simulink model "trim_sim"  (R2020b)
settings: Solver=VariableStepAuto  StartTime=0.0  StopTime=10.0  RelTol=1e-3  SampleTimeConstraint=STIndependent
undefined symbols (not defined in the file): Aircraft, Earth, Env, InitCond, WGS84
libraries: aerolibconvert2 x6, aerolibadyn x3, aerolibasang x3, aerolibatmos2 x1, sharedutil x1, aerolibbdyn x1, shared6dof x1, simulink x1, aerolibtransform2 x1, aerolibgravity2 x1
settings Model: Creator=brian  LastModifiedBy=brian

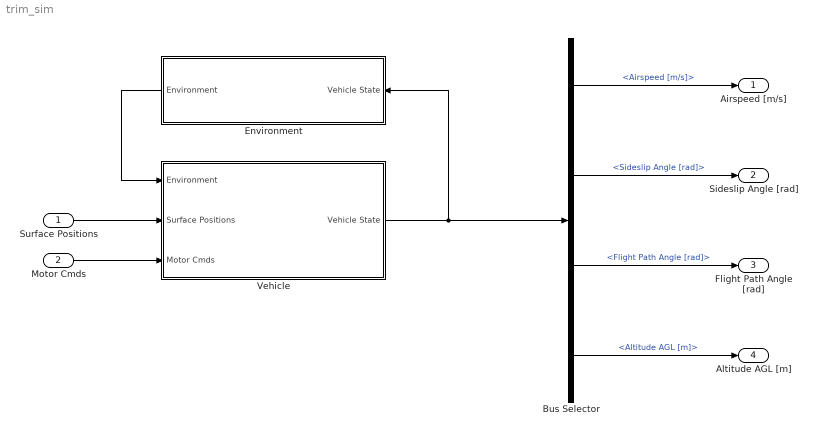
== system trim_sim ==
  Surface Positions : Inport
  Motor Cmds : Inport  Port=2  PortDimensions=Aircraft.Motor.nMotor
  Bus Selector : BusSelector  OutputSignals=Airspeed [m/s],Sideslip Angle [rad],Flight Path Angle [rad],Altitude AGL [m]
  Environment : Subsystem
  Vehicle : Subsystem
  Airspeed [m/s] : Outport
  Sideslip Angle [rad] : Outport  Port=2
  Flight Path Angle [rad] : Outport  Port=3
  Altitude AGL [m] : Outport  Port=4
  wires:
  Vehicle/1(Vehicle State) -> Environment/1(Vehicle State), Bus Selector/1
  Environment/1(Environment) -> Vehicle/1(Environment)
  Surface Positions/1 -> Vehicle/2(Surface Positions)
  Motor Cmds/1 -> Vehicle/3(Motor Cmds)
  Bus Selector/1 -> Airspeed [m/s]/1  "<Airspeed [m/s]>"
  Bus Selector/2 -> Sideslip Angle [rad]/1  "<Sideslip Angle [rad]>"
  Bus Selector/3 -> Flight Path Angle [rad]/1  "<Flight Path Angle [rad]>"
  Bus Selector/4 -> Altitude AGL [m]/1  "<Altitude AGL [m]>"

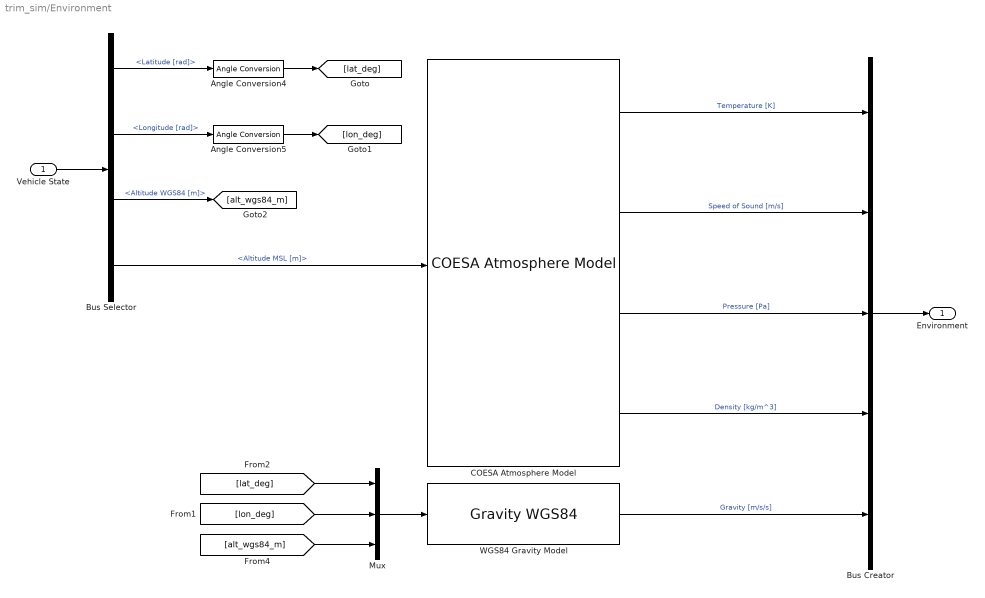
== system trim_sim/Environment ==
  Vehicle State : Inport
  Angle Conversion4 : aerolibconvert2/Angle Conversion  IU=rad  OU=deg
  Angle Conversion5 : aerolibconvert2/Angle Conversion  IU=rad  OU=deg
  Bus Creator : BusCreator  Inputs=5
  Bus Selector : BusSelector  OutputSignals=Latitude [rad],Longitude [rad],Altitude WGS84 [m],Altitude MSL [m]
  COESA Atmosphere Model : aerolibatmos2/COESA Atmosphere Model  units=Metric (MKS)  spec=1976 COESA-extended U.S. Standard Atmosphere  model=Profile  profile_var=High temperature  profile_percent=1%  profile_alt=5 km (16404 ft)  envelope_var=High temperature  envelope_percent=1%  action=Warning
  Mux : Mux  Inputs=3
  "WGS84 Gravity Model  " : GravityWGS84
  Environment : Outport
  wires:
  Vehicle State/1 -> Bus Selector/1
  Bus Selector/1 -> Angle Conversion4/1  "<Latitude [rad]>"
  Bus Selector/2 -> Angle Conversion5/1  "<Longitude [rad]>"
  Bus Selector/3 -> [alt_wgs84_m]  "<Altitude WGS84 [m]>"
  Bus Creator/1 -> Environment/1
  COESA Atmosphere Model/3 -> Bus Creator/3  "Pressure [Pa]"
  COESA Atmosphere Model/2 -> Bus Creator/2  "Speed of Sound [m/s]"
  COESA Atmosphere Model/1 -> Bus Creator/1  "Temperature [K]"
  COESA Atmosphere Model/4 -> Bus Creator/4  "Density [kg/m^3]"
  "WGS84 Gravity Model  "/1 -> Bus Creator/5  "Gravity [m/s/s]"
  Bus Selector/4 -> COESA Atmosphere Model/1  "<Altitude MSL [m]>"
  Mux/1 -> "WGS84 Gravity Model  "/1
  Angle Conversion4/1 -> [lat_deg]
  Angle Conversion5/1 -> [lon_deg]
  [alt_wgs84_m] -> Mux/3
  [lon_deg] -> Mux/2
  [lat_deg] -> Mux/1

== system trim_sim/Vehicle ==
  Environment : Inport
  Surface Positions : Inport  Port=2  PortDimensions=Aircraft.Surf.nSurf
  Motor Cmds : Inport  Port=3
  Bus Creator : BusCreator  Inputs=25
  Bus Selector : BusSelector  OutputSignals=Gravity [m/s/s],Density [kg/m^3],Speed of Sound [m/s]
  Bus Selector1 : BusSelector  OutputSignals=Body Velocity [m/s],Body Rotational Rate [rad/s],Dynamic Pressure [Pa],Airspeed [m/s],Angle of Attack [rad],Sideslip Angle [rad],DCM_be
  Forces and Moments : Subsystem
  Vehicle Model : Subsystem
  Vehicle State : Outport
  wires:
  Surface Positions/1 -> Forces and Moments/8(Surface Positions [rad])
  Environment/1 -> Bus Selector/1
  Bus Creator/1 -> Bus Selector1/1, Vehicle State/1
  Motor Cmds/1 -> Forces and Moments/9(Motor Cmds)
  Vehicle Model/1(Latitude [rad]) -> Bus Creator/1  "Latitude [rad]"
  Vehicle Model/2(Longitude [rad]) -> Bus Creator/2  "Longitude [rad]"
  Vehicle Model/3(Altitude WGS84 [m]) -> Bus Creator/3  "Altitude WGS84 [m]"
  Vehicle Model/4(Altitude MSL [m]) -> Bus Creator/4  "Altitude MSL [m]"
  Vehicle Model/5(Altitude AGL [m]) -> Bus Creator/5  "Altitude AGL [m]"
  Vehicle Model/6(NED Position [m]) -> Bus Creator/6  "NED Position [m]"
  Vehicle Model/7(NED Velocity [m/s]) -> Bus Creator/7  "NED Velocity [m/s]"
  Vehicle Model/8(NED Accel [m/s/s]) -> Bus Creator/8  "NED Accel [m/s/s]"
  Vehicle Model/9(Pitch [rad]) -> Bus Creator/9  "Pitch [rad]"
  Vehicle Model/10(Roll [rad]) -> Bus Creator/10  "Roll [rad]"
  Vehicle Model/11(Yaw [rad]) -> Bus Creator/11  "Yaw [rad]"
  Vehicle Model/12(Body Velocity [m/s]) -> Bus Creator/12  "Body Velocity [m/s]"
  Vehicle Model/13(Body Accel [m/s/s]) -> Bus Creator/13  "Body Accel [m/s/s]"
  Vehicle Model/14(Body Rotational Rate [rad/s]) -> Bus Creator/14  "Body Rotational Rate [rad/s]"
  Vehicle Model/15(Body Rotational Accel [rad/s/s]) -> Bus Creator/15  "Body Rotational Accel [rad/s/s]"
  Vehicle Model/16(Dynamic Pressure [Pa]) -> Bus Creator/16  "Dynamic Pressure [Pa]"
  Vehicle Model/17(Airspeed [m/s]) -> Bus Creator/17  "Airspeed [m/s]"
  Vehicle Model/18(Mach) -> Bus Creator/18  "Mach"
  Vehicle Model/19(Angle of Attack [rad]) -> Bus Creator/19  "Angle of Attack [rad]"
  Vehicle Model/20(Angle of Attack Rate [rad/s]) -> Bus Creator/20  "Angle of Attack Rate [rad/s]"
  Vehicle Model/21(Sideslip Angle [rad]) -> Bus Creator/21  "Sideslip Angle [rad]"
  Vehicle Model/22(Sideslip Angle Rate [rad/s]) -> Bus Creator/22  "Sideslip Angle Rate [rad/s]"
  Vehicle Model/23(Ground Track [rad]) -> Bus Creator/23  "Ground Track [rad]"
  Vehicle Model/24(Flight Path Angle [rad]) -> Bus Creator/24  "Flight Path Angle [rad]"
  Vehicle Model/25(DCM_be) -> Bus Creator/25  "DCM_be"
  Bus Selector1/7 -> Forces and Moments/7(DCM_be)  "<DCM_be>"
  Bus Selector1/6 -> Forces and Moments/6(Sideslip Angle [rad])  "<Sideslip Angle [rad]>"
  Bus Selector1/5 -> Forces and Moments/5(Angle of Attack [rad])  "<Angle of Attack [rad]>"
  Bus Selector1/4 -> Forces and Moments/4(Airspeed [m/s])  "<Airspeed [m/s]>"
  Bus Selector1/3 -> Forces and Moments/3(Dynamic Pressure [Pa])  "<Dynamic Pressure [Pa]>"
  Bus Selector1/2 -> Forces and Moments/2(Body Rotational Rate [rad/s])  "<Body Rotational Rate [rad/s]>"
  Bus Selector1/1 -> Forces and Moments/1(Body Velocity [m/s])  "<Body Velocity [m/s]>"
  Bus Selector/1 -> Forces and Moments/10(Gravity [m/s/s])  "<Gravity [m/s/s]>"
  Bus Selector/2 -> Forces and Moments/11(Density [kg/m^3]), Vehicle Model/3(Density [kg/m^3])  "<Density [kg/m^3]>"
  Bus Selector/3 -> Vehicle Model/4(Speed of Sound [m/s])  "<Speed of Sound [m/s]>"
  Forces and Moments/1(Fxyz [N]) -> Vehicle Model/1(Fxyz [N])
  Forces and Moments/2(Mxyz [N-m]) -> Vehicle Model/2(Mxyz [N-m])

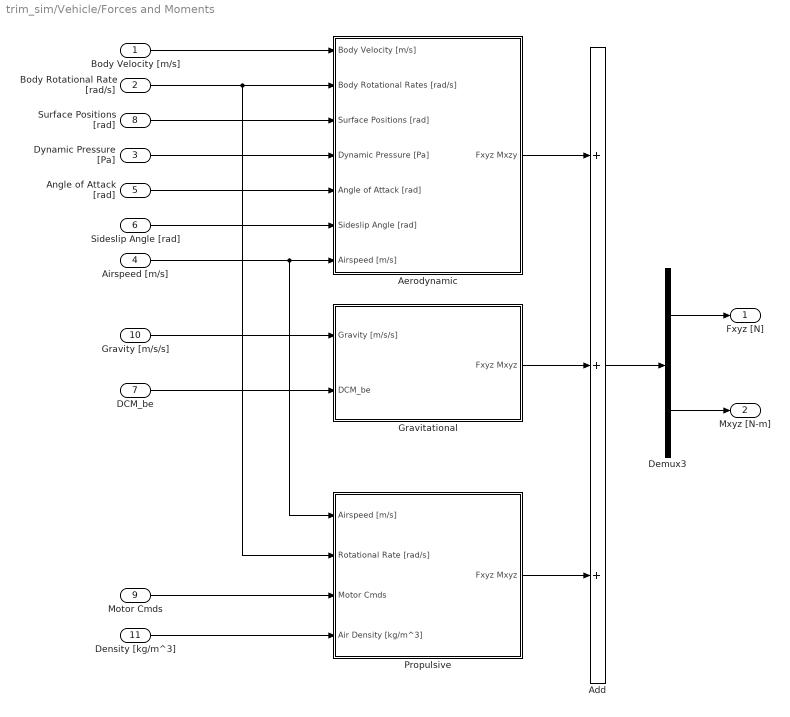
== system trim_sim/Vehicle/Forces and Moments ==
  Body Velocity [m/s] : Inport
  Body Rotational Rate [rad/s] : Inport  Port=2
  Dynamic Pressure [Pa] : Inport  Port=3
  Airspeed [m/s] : Inport  Port=4
  Angle of Attack [rad] : Inport  Port=5
  Sideslip Angle [rad] : Inport  Port=6
  DCM_be : Inport  Port=7
  Surface Positions [rad] : Inport  Port=8
  Motor Cmds : Inport  Port=9
  Gravity [m/s/s] : Inport  Port=10
  Density [kg/m^3] : Inport  Port=11
  Add : Sum  Inputs=+++
  Aerodynamic : Subsystem
  Demux3 : Demux  Outputs=2
  Gravitational : Subsystem
  Propulsive : Subsystem
  Fxyz [N] : Outport
  Mxyz [N-m] : Outport  Port=2
  wires:
  Propulsive/1(Fxyz Mxyz) -> Add/3
  Density [kg/m^3]/1 -> Propulsive/4(Air Density [kg/m^3])
  Motor Cmds/1 -> Propulsive/3(Motor Cmds)
  Add/1 -> Demux3/1
  Demux3/2 -> Mxyz [N-m]/1
  Aerodynamic/1(Fxyz Mxzy) -> Add/1
  Demux3/1 -> Fxyz [N]/1
  Body Rotational Rate [rad/s]/1 -> Propulsive/2(Rotational Rate [rad/s]), Aerodynamic/2(Body Rotational Rates [rad/s])
  DCM_be/1 -> Gravitational/2(DCM_be)
  Angle of Attack [rad]/1 -> Aerodynamic/5(Angle of Attack [rad])
  Gravitational/1(Fxyz Mxyz) -> Add/2
  Sideslip Angle [rad]/1 -> Aerodynamic/6(Sideslip Angle [rad])
  Body Velocity [m/s]/1 -> Aerodynamic/1(Body Velocity [m/s])
  Dynamic Pressure [Pa]/1 -> Aerodynamic/4(Dynamic Pressure [Pa])
  Airspeed [m/s]/1 -> Propulsive/1(Airspeed [m/s]), Aerodynamic/7(Airspeed [m/s])
  Gravity [m/s/s]/1 -> Gravitational/1(Gravity [m/s/s])
  Surface Positions [rad]/1 -> Aerodynamic/3(Surface Positions [rad])

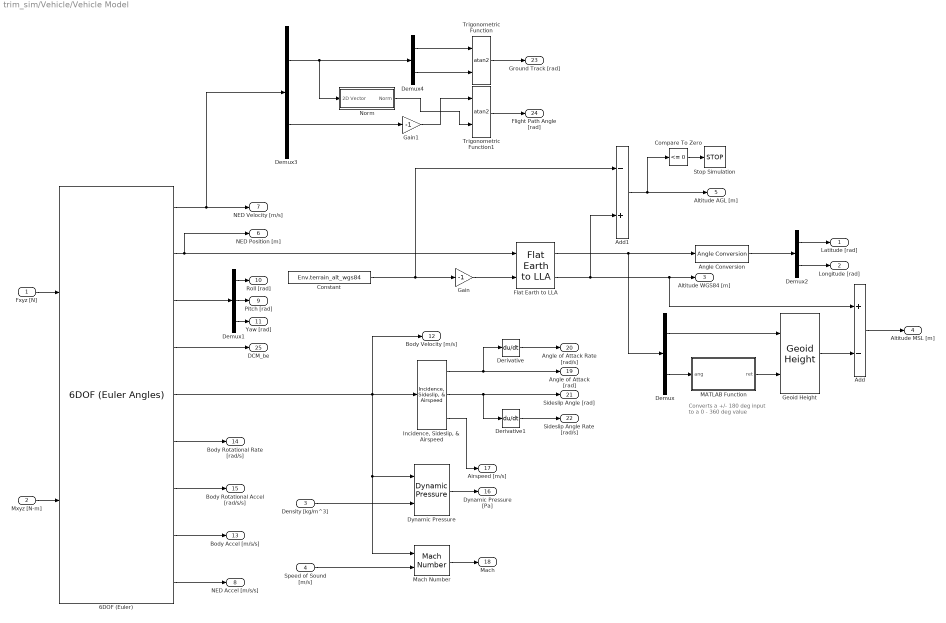
== system trim_sim/Vehicle/Vehicle Model ==
  note: Converts a +/- 180 deg
      | input to a 0 - 360 deg value
  Fxyz [N] : Inport
  Mxyz [N-m] : Inport  Port=2
  Density [kg/m^3] : Inport  Port=3
  Speed of Sound [m/s] : Inport  Port=4
  6DOF (Euler) : shared6dof/6DOF (Euler Angles)  units=Metric (MKS)  mtype=Fixed  rep=Euler Angles  xme_0=InitCond.ned_pos_m  Vm_0=InitCond.body_vel_mps  eul_0=InitCond.euler_rad  pm_0=InitCond.body_rot_rate_radps  mass_0=Aircraft.Mass.mass_kg  mass_e=0.5  mass_f=2.0  inertia=Aircraft.Mass.inertia_kgm2  inertia_e=eye(3)  inertia_f=2*eye(3)  k_quat=1.0  vre_flag=on  abi_flag=on  aMode=0  xme_statename=''  Vm_statename=''  eul_statename=''  quat_statename=''  pm_statename=''  mass_statename=''
      settings: SourceProductBaseCode=AE,PW,MT,UV,VE,VP
  Add : Sum  Inputs=+-
  Add1 : Sum  Inputs=-+
  Angle Conversion : aerolibconvert2/Angle Conversion  IU=deg  OU=rad
  Compare To Zero : simulink/Logic and Bit Operations/Compare To Zero  relop=<=  OutDataTypeStr=boolean
  Constant : Constant  Value=Env.terrain_alt_wgs84
  Demux : Demux  Outputs=2
  Demux1 : Demux  Outputs=3
  Demux2 : Demux  Outputs=2
  Demux3 : Demux  Outputs=[2 1]
  Demux4 : Demux  Outputs=2
  Derivative : Derivative
  Derivative1 : Derivative
  Dynamic Pressure : aerolibasang/Dynamic Pressure
  Flat Earth to LLA : aerolibtransform2/Flat Earth to LLA  units=Metric (MKS)  ptype=Earth (WGS84)  F=1/298.257223563  R=6378137  refPosPort=off  LL0=[rad2deg(InitCond.lat_rad) rad2deg(InitCond.lon_rad)]  psi=0
  Gain : Gain  Gain=-1
  Gain1 : Gain  Gain=-1
  Geoid Height : aerolibgravity2/Geoid Height  units=Metric (MKS)  gtype=EGM2008  datafile='geoidegm96grid'  dtype=double  action=Warning
      settings: SourceProductBaseCode=AE
  "Incidence, Sideslip, & Airspeed" : aerolibasang/Incidence, Sideslip, & Airspeed
  MATLAB Function : MATLAB Function  TreatAsAtomicUnit=on
  Mach Number : aerolibasang/Mach Number
      settings: SourceProductBaseCode=AE
  Norm : Subsystem
  Stop Simulation : Stop
  Trigonometric Function : Trigonometry  Operator=atan2
  Trigonometric Function1 : Trigonometry  Operator=atan2
  Latitude [rad] : Outport
  Longitude [rad] : Outport  Port=2
  Altitude WGS84 [m] : Outport  Port=3
  Altitude MSL [m] : Outport  Port=4
  Altitude AGL [m] : Outport  Port=5
  NED Position [m] : Outport  Port=6
  NED Velocity [m/s] : Outport  Port=7
  NED Accel [m/s/s] : Outport  Port=8
  Pitch [rad] : Outport  Port=9
  Roll [rad] : Outport  Port=10
  Yaw [rad] : Outport  Port=11
  Body Velocity [m/s] : Outport  Port=12
  Body Accel [m/s/s] : Outport  Port=13
  Body Rotational Rate [rad/s] : Outport  Port=14
  Body Rotational Accel [rad/s/s] : Outport  Port=15
  Dynamic Pressure [Pa] : Outport  Port=16
  Airspeed [m/s] : Outport  Port=17
  Mach : Outport  Port=18
  Angle of Attack [rad] : Outport  Port=19
  Angle of Attack Rate [rad/s] : Outport  Port=20
  Sideslip Angle [rad] : Outport  Port=21
  Sideslip Angle Rate [rad/s] : Outport  Port=22
  Ground Track [rad] : Outport  Port=23
  Flight Path Angle [rad] : Outport  Port=24
  DCM_be : Outport  Port=25
  wires:
  Fxyz [N]/1 -> 6DOF (Euler)/1
  Mxyz [N-m]/1 -> 6DOF (Euler)/2
  6DOF (Euler)/5 -> Body Velocity [m/s]/1, "Incidence, Sideslip, & Airspeed"/1, Dynamic Pressure/1, Mach Number/1
  Flat Earth to LLA/1 -> Demux/1, Angle Conversion/1
  Flat Earth to LLA/2 -> Add1/2, Add/1, Altitude WGS84 [m]/1
  Geoid Height/1 -> Add/2
  Demux/2 -> MATLAB Function/1(ang)
  Demux/1 -> Geoid Height/1
  "Incidence, Sideslip, & Airspeed"/3 -> Airspeed [m/s]/1
  Density [kg/m^3]/1 -> Dynamic Pressure/2
  Angle Conversion/1 -> Demux2/1
  6DOF (Euler)/4 -> DCM_be/1
  Demux1/1 -> Roll [rad]/1
  6DOF (Euler)/3 -> Demux1/1
  Demux1/2 -> Pitch [rad]/1
  Demux1/3 -> Yaw [rad]/1
  Dynamic Pressure/1 -> Dynamic Pressure [Pa]/1
  "Incidence, Sideslip, & Airspeed"/1 -> Derivative/1, Angle of Attack [rad]/1
  "Incidence, Sideslip, & Airspeed"/2 -> Derivative1/1, Sideslip Angle [rad]/1
  Add/1 -> Altitude MSL [m]/1
  Gain/1 -> Flat Earth to LLA/2
  Demux2/2 -> Longitude [rad]/1
  Demux2/1 -> Latitude [rad]/1
  6DOF (Euler)/2 -> NED Position [m]/1, Flat Earth to LLA/1
  6DOF (Euler)/6 -> Body Rotational Rate [rad/s]/1
  6DOF (Euler)/7 -> Body Rotational Accel [rad/s/s]/1
  6DOF (Euler)/8 -> Body Accel [m/s/s]/1
  6DOF (Euler)/1 -> Demux3/1, NED Velocity [m/s]/1
  MATLAB Function/1(ret) -> Geoid Height/2
  Demux3/1 -> Norm/1(2D Vector), Demux4/1
  Demux4/1 -> Trigonometric Function/1
  Demux4/2 -> Trigonometric Function/2
  Trigonometric Function/1 -> Ground Track [rad]/1
  Demux3/2 -> Gain1/1
  Gain1/1 -> Trigonometric Function1/1
  Norm/1(Norm) -> Trigonometric Function1/2
  Trigonometric Function1/1 -> Flight Path Angle [rad]/1
  6DOF (Euler)/9 -> NED Accel [m/s/s]/1
  Speed of Sound [m/s]/1 -> Mach Number/2
  Mach Number/1 -> Mach/1
  Derivative/1 -> Angle of Attack Rate [rad/s]/1
  Derivative1/1 -> Sideslip Angle Rate [rad/s]/1
  Constant/1 -> Add1/1, Gain/1
  Add1/1 -> Compare To Zero/1, Altitude AGL [m]/1
  Compare To Zero/1 -> Stop Simulation/1

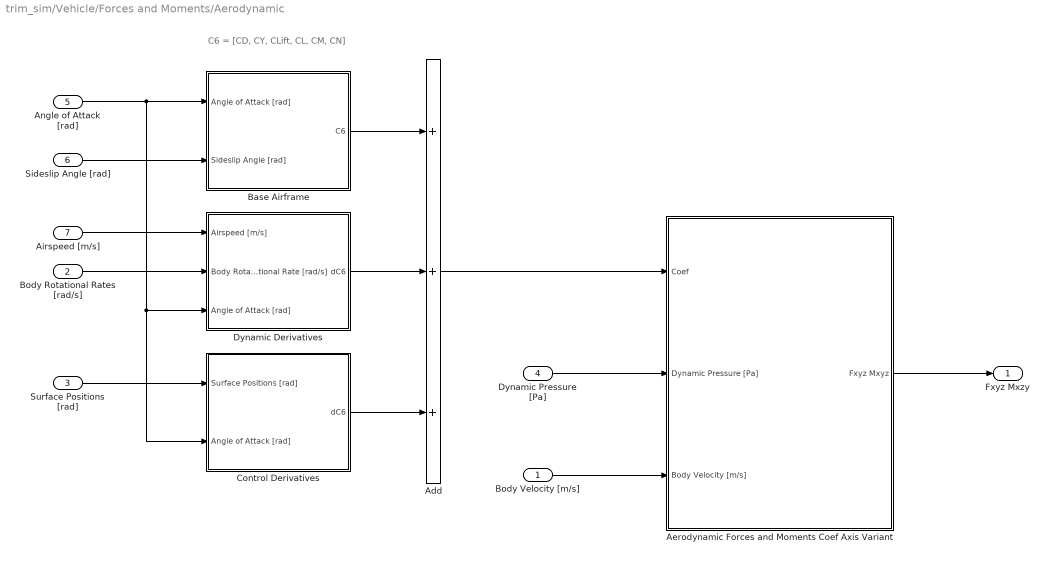
== system trim_sim/Vehicle/Forces and Moments/Aerodynamic ==
  note: C6 = [CD, CY, CLift, CL, CM, CN]
  Body Velocity [m/s] : Inport
  Body Rotational Rates [rad/s] : Inport  Port=2
  Surface Positions [rad] : Inport  Port=3
  Dynamic Pressure [Pa] : Inport  Port=4
  Angle of Attack [rad] : Inport  Port=5
  Sideslip Angle [rad] : Inport  Port=6
  Airspeed [m/s] : Inport  Port=7
  Add : Sum  Inputs=+++
  Aerodynamic Forces and Moments Coef Axis Variant : Subsystem  Variant=on
  Base Airframe : Subsystem
  Control Derivatives : Subsystem
  Dynamic Derivatives : Subsystem
  Fxyz Mxzy : Outport
  wires:
  Base Airframe/1(C6) -> Add/1
  Dynamic Derivatives/1(dC6) -> Add/2
  Sideslip Angle [rad]/1 -> Base Airframe/2(Sideslip Angle [rad])
  Angle of Attack [rad]/1 -> Base Airframe/1(Angle of Attack [rad]), Control Derivatives/2(Angle of Attack [rad]), Dynamic Derivatives/3(Angle of Attack [rad])
  Body Rotational Rates [rad/s]/1 -> Dynamic Derivatives/2(Body Rotational Rate [rad/s])
  Airspeed [m/s]/1 -> Dynamic Derivatives/1(Airspeed [m/s])
  Surface Positions [rad]/1 -> Control Derivatives/1(Surface Positions [rad])
  Control Derivatives/1(dC6) -> Add/3
  Add/1 -> Aerodynamic Forces and Moments Coef Axis Variant/1(Coef)
  Body Velocity [m/s]/1 -> Aerodynamic Forces and Moments Coef Axis Variant/3(Body Velocity [m/s])
  Dynamic Pressure [Pa]/1 -> Aerodynamic Forces and Moments Coef Axis Variant/2(Dynamic Pressure [Pa])
  Aerodynamic Forces and Moments Coef Axis Variant/1(Fxyz Mxyz) -> Fxyz Mxzy/1

== system trim_sim/Vehicle/Forces and Moments/Gravitational ==
  Gravity [m/s/s] : Inport
  DCM_be : Inport  Port=2
  Gravity Moment : Constant  Value=[0 0 0]
  Mux : Mux  Inputs=2
  Product : Product
  Product1 : Product  Multiplication=Matrix(*)
  Reshape : Reshape  OutputDimensionality=Column vector (2-D)
  Reshape1 : Reshape
  UAV Mass : Constant  Value=Aircraft.Mass.mass_kg
  Fxyz Mxyz : Outport
  wires:
  UAV Mass/1 -> Product/2
  Product/1 -> Product1/2  "Gravity Force NED [N]"
  DCM_be/1 -> Product1/1
  Gravity Moment/1 -> Mux/2
  Mux/1 -> Fxyz Mxyz/1
  Reshape/1 -> Product/1
  Gravity [m/s/s]/1 -> Reshape/1
  Reshape1/1 -> Mux/1
  Product1/1 -> Reshape1/1  "Gravity Force Body [N]"

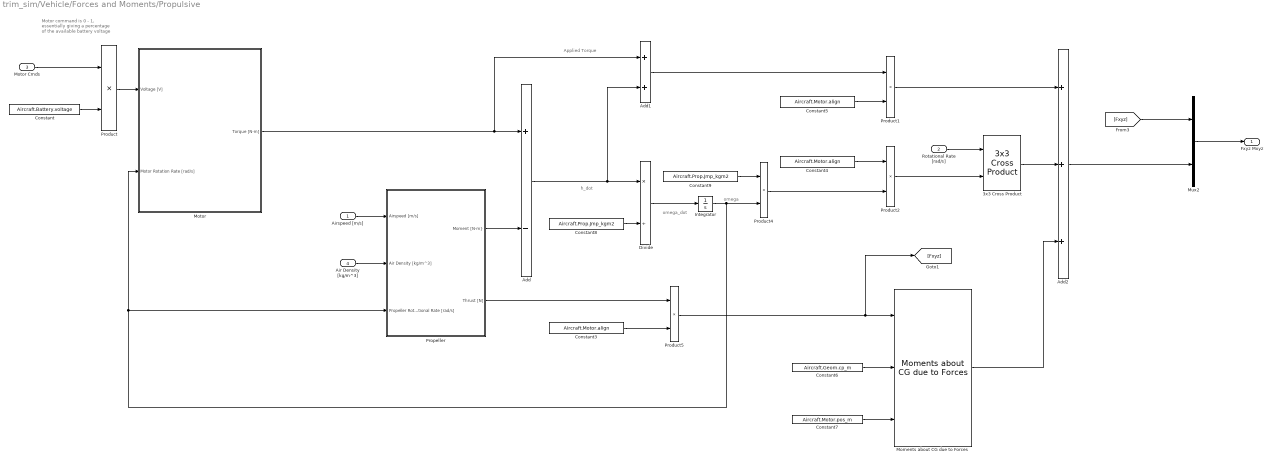
== system trim_sim/Vehicle/Forces and Moments/Propulsive ==
  note: Applied Torque
  note: omega
  note: Motor command is 0 - 1,
      | essentially giving a percentage
      | of the available battery voltage
  note: omega_dot
  note: h_dot
  Airspeed [m/s] : Inport
  Rotational Rate [rad/s] : Inport  Port=2
  Motor Cmds : Inport  Port=3
  Air Density [kg/m^3] : Inport  Port=4
  3x3 Cross Product : sharedutil/3x3 Cross Product  aMode=aMode
      settings: SourceProductBaseCode=AE,PW,MT,UV,VE,VP
  Add : Sum  Inputs=+-
  Add1 : Sum
  Add2 : Sum  Inputs=+++
  Constant : Constant  Value=Aircraft.Battery.voltage
  Constant3 : Constant  Value=Aircraft.Motor.align
  Constant4 : Constant  Value=Aircraft.Motor.align
  Constant5 : Constant  Value=Aircraft.Motor.align
  Constant6 : Constant  Value=Aircraft.Geom.cp_m
  Constant7 : Constant  Value=Aircraft.Motor.pos_m
  Constant8 : Constant  Value=Aircraft.Prop.Jmp_kgm2
  Constant9 : Constant  Value=Aircraft.Prop.Jmp_kgm2
  Divide : Product  Inputs=*/
  Integrator : Integrator  InitialCondition=InitCond.engine_speed_radps
  Moments about CG due to Forces : aerolibbdyn/Moments about CG  due to Forces
      settings: SourceProductBaseCode=AE
  Motor : Subsystem
  Mux2 : Mux  Inputs=2
  Product{,1..2,4..5} (5 alike) : Product
  Propeller : Subsystem
  Fxyz Mxyz : Outport
  wires:
  Divide/1 -> Integrator/1
  Constant3/1 -> Product5/2
  Constant8/1 -> Divide/2
  Product5/1 -> [Fxyz], Moments about CG due to Forces/1
  Product2/1 -> 3x3 Cross Product/2
  Product4/1 -> Product2/2
  Air Density [kg/m^3]/1 -> Propeller/2(Air Density [kg/m^3])
  Rotational Rate [rad/s]/1 -> 3x3 Cross Product/1
  Constant6/1 -> Moments about CG due to Forces/2
  Add/1 -> Add1/2, Divide/1
  Constant/1 -> Product/2
  Constant7/1 -> Moments about CG due to Forces/3
  Add1/1 -> Product1/1
  Product/1 -> Motor/1(Voltage [V])
  Constant5/1 -> Product1/2
  Propeller/2(Thrust [N]) -> Product5/1
  Integrator/1 -> Product4/2, Propeller/3(Propeller Rotational Rate [rad/s]), Motor/2(Motor Rotation Rate [rad/s])
  Airspeed [m/s]/1 -> Propeller/1(Airspeed [m/s])
  Moments about CG due to Forces/1 -> Add2/3
  Add2/1 -> Mux2/2
  3x3 Cross Product/1 -> Add2/2
  Mux2/1 -> Fxyz Mxyz/1
  Motor Cmds/1 -> Product/1
  [Fxyz] -> Mux2/1
  Propeller/1("Moment [N-m}") -> Add/2
  Constant4/1 -> Product2/1
  Motor/1(Torque [N-m]) -> Add1/1, Add/1
  Product1/1 -> Add2/1
  Constant9/1 -> Product4/1

== system trim_sim/Vehicle/Vehicle Model/Norm ==
  2D Vector : Inport
  Product : Product
  Sqrt : Sqrt  SaturateOnIntegerOverflow=on
  Sum of Elements : Sum  Inputs=+
  Norm : Outport
  wires:
  2D Vector/1 -> Product/2, Product/1
  Product/1 -> Sum of Elements/1
  Sum of Elements/1 -> Sqrt/1
  Sqrt/1 -> Norm/1

== system trim_sim/Vehicle/Forces and Moments/Aerodynamic/Aerodynamic Forces and Moments Coef Axis Variant ==
  Coef : Inport
  Dynamic Pressure [Pa] : Inport  Port=2
  Body Velocity [m/s] : Inport  Port=3
  Body Axis Coef : Subsystem  VariantControl=Aircraft.Aero.axis == 3
  Stability Axis Coef : Subsystem  VariantControl=Aircraft.Aero.axis == 2
  Wind Axis Coef : Subsystem  VariantControl=Aircraft.Aero.axis == 1
  Fxyz Mxyz : Outport

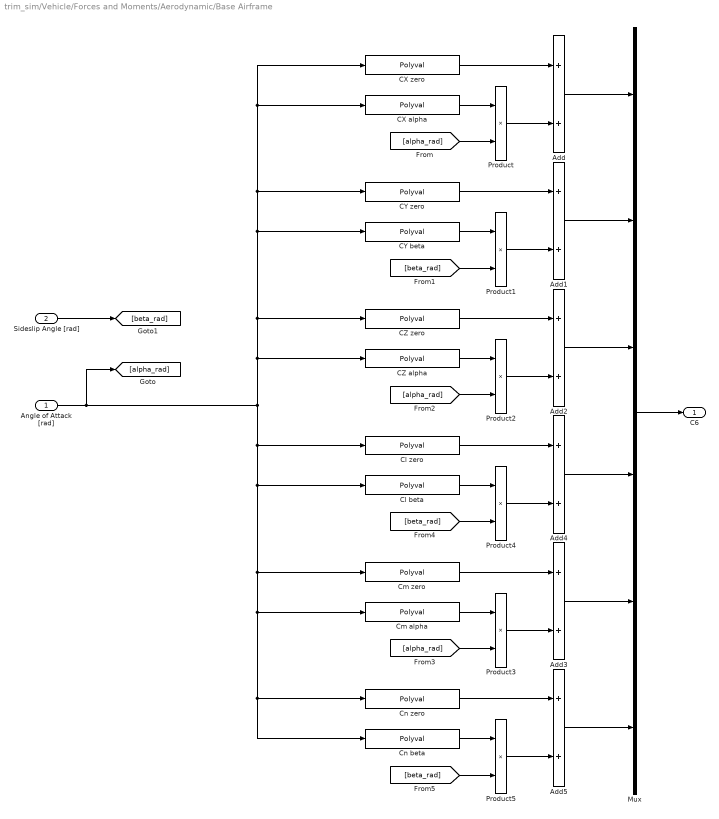
== system trim_sim/Vehicle/Forces and Moments/Aerodynamic/Base Airframe ==
  Angle of Attack [rad] : Inport
  Sideslip Angle [rad] : Inport  Port=2
  Add{,1..5} (6 alike) : Sum
  CX alpha : Polyval  Coefs=Aircraft.Aero.CX.alpha
  CX zero : Polyval  Coefs=Aircraft.Aero.CX.zero
  CY beta : Polyval  Coefs=Aircraft.Aero.CY.beta
  CY zero : Polyval  Coefs=Aircraft.Aero.CY.zero
  CZ alpha : Polyval  Coefs=Aircraft.Aero.CZ.alpha
  CZ zero : Polyval  Coefs=Aircraft.Aero.CZ.zero
  Cl beta : Polyval  Coefs=Aircraft.Aero.Cl.beta
  Cl zero : Polyval  Coefs=Aircraft.Aero.Cl.zero
  Cm alpha : Polyval  Coefs=Aircraft.Aero.Cm.alpha
  Cm zero : Polyval  Coefs=Aircraft.Aero.Cm.zero
  Cn beta : Polyval  Coefs=Aircraft.Aero.Cn.beta
  Cn zero : Polyval  Coefs=Aircraft.Aero.Cn.zero
  Mux : Mux  Inputs=6
  Product{,1..5} (6 alike) : Product
  C6 : Outport
  wires:
  Product/1 -> Add/2
  Add/1 -> Mux/1
  CX alpha/1 -> Product/1
  CX zero/1 -> Add/1
  Sideslip Angle [rad]/1 -> [beta_rad]
  [alpha_rad] -> Product/2
  Mux/1 -> C6/1
  [beta_rad] -> Product1/2
  CY zero/1 -> Add1/1
  CY beta/1 -> Product1/1
  Product1/1 -> Add1/2
  Add1/1 -> Mux/2
  CZ zero/1 -> Add2/1
  CZ alpha/1 -> Product2/1
  Add2/1 -> Mux/3
  Product2/1 -> Add2/2
  Product3/1 -> Add3/2
  Add3/1 -> Mux/5
  Cm alpha/1 -> Product3/1
  Cm zero/1 -> Add3/1
  [alpha_rad] -> Product2/2
  [alpha_rad] -> Product3/2
  Add4/1 -> Mux/4
  Product4/1 -> Add4/2
  Cl beta/1 -> Product4/1
  Cl zero/1 -> Add4/1
  [beta_rad] -> Product4/2
  [beta_rad] -> Product5/2
  Cn zero/1 -> Add5/1
  Cn beta/1 -> Product5/1
  Product5/1 -> Add5/2
  Add5/1 -> Mux/6
  Angle of Attack [rad]/1 -> [alpha_rad], Cl zero/1, Cl beta/1, Cm zero/1, Cm alpha/1, Cn zero/1, Cn beta/1, CZ alpha/1, CZ zero/1, CY beta/1, CY zero/1, CX alpha/1, CX zero/1

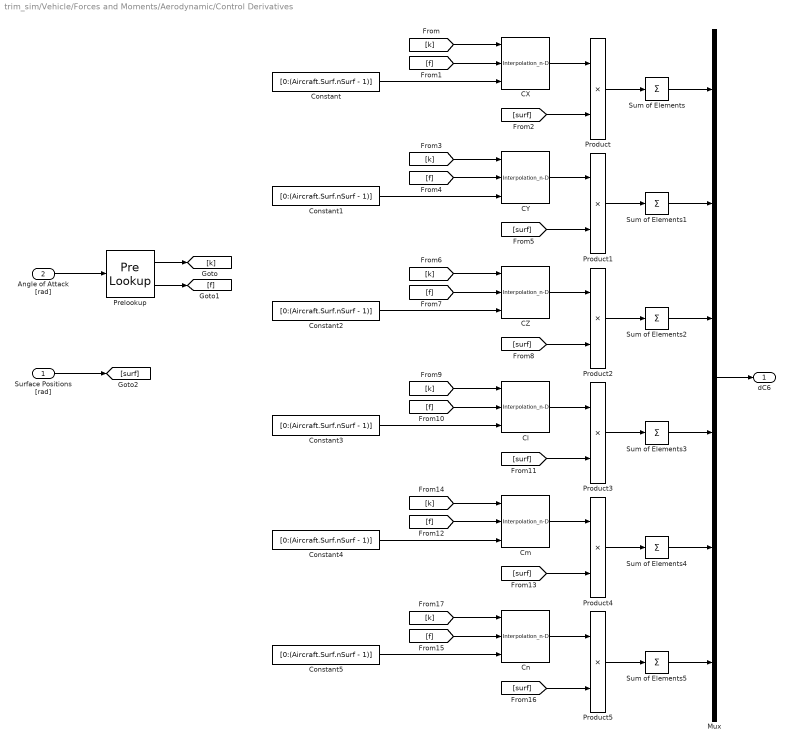
== system trim_sim/Vehicle/Forces and Moments/Aerodynamic/Control Derivatives ==
  Surface Positions [rad] : Inport
  Angle of Attack [rad] : Inport  Port=2
  CX : Interpolation_n-D  Table=Aircraft.Aero.CX.surf  DiagnosticForOutOfRangeInput=Warning  NumSelectionDims=1  InternalRulePriority=Speed
      settings: InputPortMap=u0,u1,u2
  CY : Interpolation_n-D  Table=Aircraft.Aero.CY.surf  DiagnosticForOutOfRangeInput=Warning  NumSelectionDims=1  InternalRulePriority=Speed
      settings: InputPortMap=u0,u1,u2
  CZ : Interpolation_n-D  Table=Aircraft.Aero.CZ.surf  DiagnosticForOutOfRangeInput=Warning  NumSelectionDims=1  InternalRulePriority=Speed
      settings: InputPortMap=u0,u1,u2
  Cl : Interpolation_n-D  Table=Aircraft.Aero.Cl.surf  DiagnosticForOutOfRangeInput=Warning  NumSelectionDims=1  InternalRulePriority=Speed
      settings: InputPortMap=u0,u1,u2
  Cm : Interpolation_n-D  Table=Aircraft.Aero.Cm.surf  DiagnosticForOutOfRangeInput=Warning  NumSelectionDims=1  InternalRulePriority=Speed
      settings: InputPortMap=u0,u1,u2
  Cn : Interpolation_n-D  Table=Aircraft.Aero.Cn.surf  DiagnosticForOutOfRangeInput=Warning  NumSelectionDims=1  InternalRulePriority=Speed
      settings: InputPortMap=u0,u1,u2
  Constant{,1..5} (6 alike) : Constant  Value=[0:(Aircraft.Surf.nSurf - 1)]
  Mux : Mux  Inputs=6
  Prelookup : PreLookup  BreakpointsData=Aircraft.Aero.CntrlEff.alpha  ExtrapMethod=Linear
  Product{,1..5} (6 alike) : Product
  Sum of Elements{,1..5} (6 alike) : Sum  Inputs=+
  dC6 : Outport
  wires:
  [k] -> Cm/1
  CY/1 -> Product1/1
  [f] -> Cn/2
  Product5/1 -> Sum of Elements5/1
  [surf] -> Product5/2
  Constant4/1 -> Cm/3
  Sum of Elements1/1 -> Mux/2
  [k] -> Cn/1
  Sum of Elements5/1 -> Mux/6
  Constant3/1 -> Cl/3
  [surf] -> Product3/2
  [k] -> Cl/1
  [f] -> Cl/2
  Constant2/1 -> CZ/3
  [k] -> CZ/1
  [surf] -> Product2/2
  Cl/1 -> Product3/1
  CZ/1 -> Product2/1
  Product2/1 -> Sum of Elements2/1
  Product3/1 -> Sum of Elements3/1
  Product1/1 -> Sum of Elements1/1
  Product/1 -> Sum of Elements/1
  [k] -> CY/1
  [f] -> CY/2
  Constant1/1 -> CY/3
  Constant/1 -> CX/3
  Cm/1 -> Product4/1
  [k] -> CX/1
  [surf] -> Product/2
  Prelookup/2 -> [f]
  Mux/1 -> dC6/1
  Prelookup/1 -> [k]
  Product4/1 -> Sum of Elements4/1
  Cn/1 -> Product5/1
  Angle of Attack [rad]/1 -> Prelookup/1
  Surface Positions [rad]/1 -> [surf]
  [f] -> CZ/2
  [f] -> Cm/2
  Sum of Elements2/1 -> Mux/3
  CX/1 -> Product/1
  [f] -> CX/2
  Constant5/1 -> Cn/3
  [surf] -> Product4/2
  Sum of Elements/1 -> Mux/1
  Sum of Elements4/1 -> Mux/5
  [surf] -> Product1/2
  Sum of Elements3/1 -> Mux/4

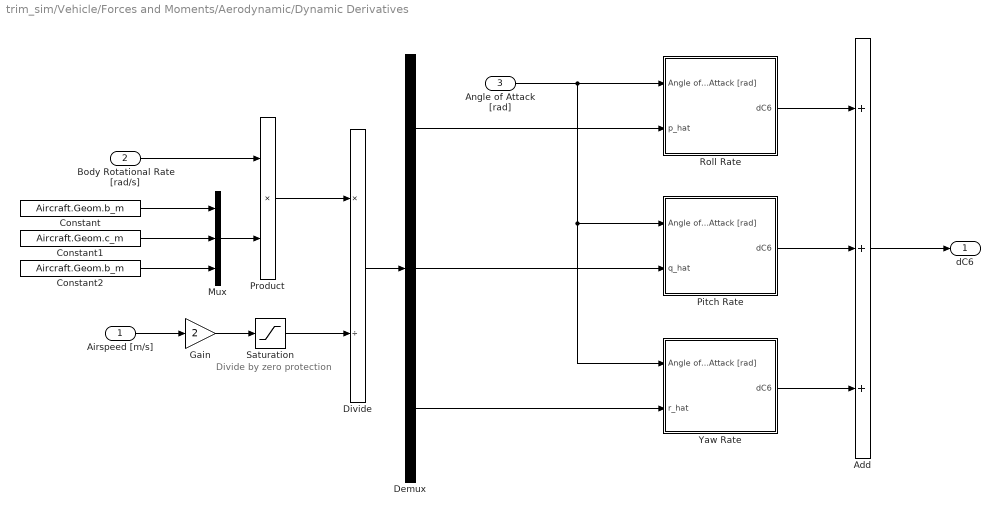
== system trim_sim/Vehicle/Forces and Moments/Aerodynamic/Dynamic Derivatives ==
  note: Divide by zero protection
  Airspeed [m/s] : Inport
  Body Rotational Rate [rad/s] : Inport  Port=2
  Angle of Attack [rad] : Inport  Port=3
  Add : Sum  Inputs=+++
  Constant : Constant  Value=Aircraft.Geom.b_m
  Constant1 : Constant  Value=Aircraft.Geom.c_m
  Constant2 : Constant  Value=Aircraft.Geom.b_m
  Demux : Demux  Outputs=3
  Divide : Product  Inputs=*/
  Gain : Gain  Gain=2
  Mux : Mux  Inputs=3
  Pitch Rate : Subsystem
  Product : Product
  Roll Rate : Subsystem
  Saturation : Saturate  UpperLimit=inf  LowerLimit=1e-3
  Yaw Rate : Subsystem
  dC6 : Outport
  wires:
  Constant/1 -> Mux/1
  Body Rotational Rate [rad/s]/1 -> Product/1
  Mux/1 -> Product/2
  Airspeed [m/s]/1 -> Gain/1
  Gain/1 -> Saturation/1
  Product/1 -> Divide/1
  Saturation/1 -> Divide/2
  Divide/1 -> Demux/1
  Demux/1 -> Roll Rate/2(p_hat)
  Demux/2 -> Pitch Rate/2(q_hat)
  Demux/3 -> Yaw Rate/2(r_hat)
  Angle of Attack [rad]/1 -> Yaw Rate/1(Angle of Attack [rad]), Pitch Rate/1(Angle of Attack [rad]), Roll Rate/1(Angle of Attack [rad])
  Roll Rate/1(dC6) -> Add/1
  Pitch Rate/1(dC6) -> Add/2
  Yaw Rate/1(dC6) -> Add/3
  Constant2/1 -> Mux/3
  Constant1/1 -> Mux/2
  Add/1 -> dC6/1

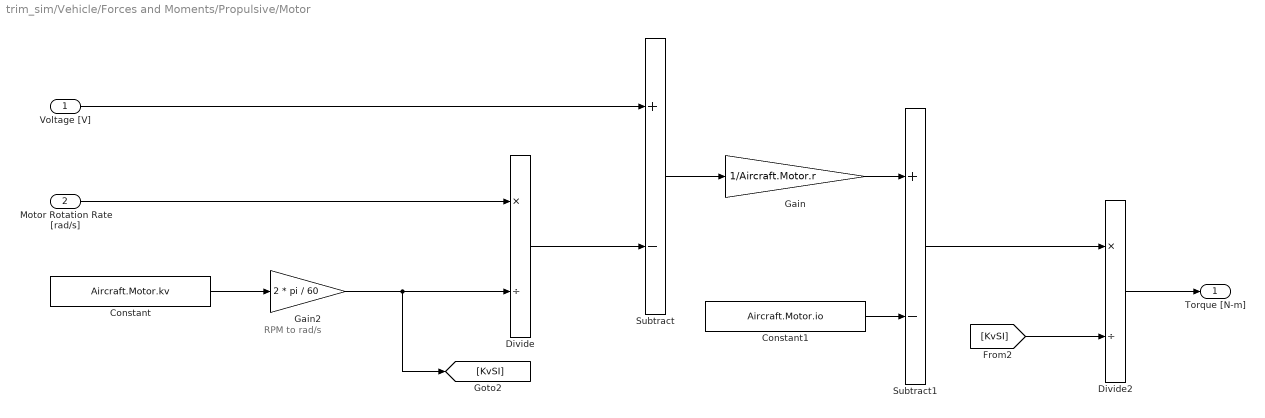
== system trim_sim/Vehicle/Forces and Moments/Propulsive/Motor ==
  note: RPM to rad/s
  Voltage [V] : Inport
  Motor Rotation Rate [rad/s] : Inport  Port=2
  Constant : Constant  Value=Aircraft.Motor.kv
  Constant1 : Constant  Value=Aircraft.Motor.io
  Divide : Product  Inputs=*/
  Divide2 : Product  Inputs=*/
  Gain : Gain  Gain=1/Aircraft.Motor.r
  Gain2 : Gain  Gain=2 * pi / 60
  Subtract : Sum  Inputs=+-
  Subtract1 : Sum  Inputs=+-
  Torque [N-m] : Outport
  wires:
  Gain2/1 -> [KvSI], Divide/2
  [KvSI] -> Divide2/2
  Constant1/1 -> Subtract1/2
  Motor Rotation Rate [rad/s]/1 -> Divide/1
  Divide/1 -> Subtract/2
  Constant/1 -> Gain2/1
  Gain/1 -> Subtract1/1
  Subtract1/1 -> Divide2/1
  Voltage [V]/1 -> Subtract/1
  Divide2/1 -> Torque [N-m]/1
  Subtract/1 -> Gain/1

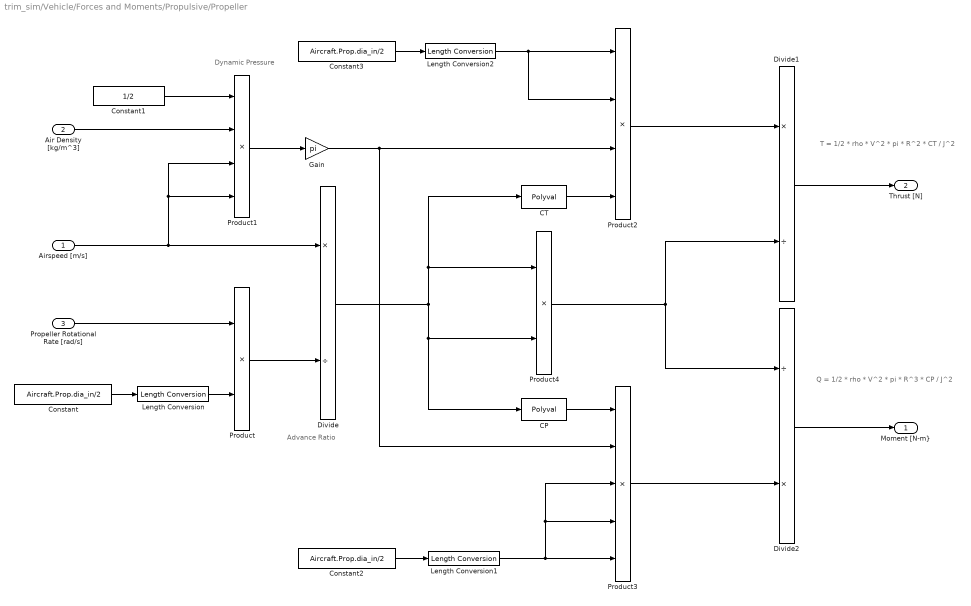
== system trim_sim/Vehicle/Forces and Moments/Propulsive/Propeller ==
  note: Dynamic Pressure
  note: Q = 1/2 * rho * V^2 * pi * R^3 * CP / J^2
  note: T = 1/2 * rho * V^2 * pi * R^2 * CT / J^2
  note: Advance Ratio
  Airspeed [m/s] : Inport
  Air Density [kg/m^3] : Inport  Port=2
  Propeller Rotational Rate [rad/s] : Inport  Port=3
  CP : Polyval  Coefs=Aircraft.prop.cp
  CT : Polyval  Coefs=Aircraft.prop.ct
  Constant : Constant  Value=Aircraft.Prop.dia_in/2
  Constant1 : Constant  Value=1/2
  Constant2 : Constant  Value=Aircraft.Prop.dia_in/2
  Constant3 : Constant  Value=Aircraft.Prop.dia_in/2
  Divide : Product  Inputs=*/
  Divide1 : Product  Inputs=*/
  Divide2 : Product  Inputs=/*
  Gain : Gain  Gain=pi
  Length Conversion : aerolibconvert2/Length Conversion  IU=in  OU=m
  Length Conversion1 : aerolibconvert2/Length Conversion  IU=in  OU=m
  Length Conversion2 : aerolibconvert2/Length Conversion  IU=in  OU=m
  Product : Product
  Product1 : Product  Inputs=4
  Product2 : Product  Inputs=4
  Product3 : Product  Inputs=5
  Product4 : Product
  "Moment [N-m}" : Outport
  Thrust [N] : Outport  Port=2
  wires:
  Divide2/1 -> "Moment [N-m}"/1
  Length Conversion/1 -> Product/2
  Product4/1 -> Divide2/1, Divide1/2
  Constant2/1 -> Length Conversion1/1
  Airspeed [m/s]/1 -> Divide/1, Product1/4, Product1/3
  Propeller Rotational Rate [rad/s]/1 -> Product/1
  Length Conversion1/1 -> Product3/4, Product3/3, Product3/5
  Product1/1 -> Gain/1
  Gain/1 -> Product3/2, Product2/3
  Air Density [kg/m^3]/1 -> Product1/2
  Divide1/1 -> Thrust [N]/1
  Product3/1 -> Divide2/2
  Constant1/1 -> Product1/1
  CP/1 -> Product3/1
  CT/1 -> Product2/4
  Product2/1 -> Divide1/1
  Length Conversion2/1 -> Product2/2, Product2/1
  Constant/1 -> Length Conversion/1
  Constant3/1 -> Length Conversion2/1
  Divide/1 -> Product4/2, CP/1, Product4/1, CT/1
  Product/1 -> Divide/2

== system trim_sim/Vehicle/Forces and Moments/Aerodynamic/Aerodynamic Forces and Moments Coef Axis Variant/Body Axis Coef ==
  Coef : Inport
  Dynamic Pressure [Pa] : Inport  Port=2
  Body Velocity [m/s] : Inport  Port=3
  "Aerodynamic Forces and Moments " : aerolibadyn/Aerodynamic Forces and Moments   inputAxes=Body  outputForceAxes=Body  outputMomentAxes=Body  S=Aircraft.Geom.s_m2  b=Aircraft.Geom.b_m  cbar=Aircraft.Geom.c_m
  Constant : Constant  Value=Aircraft.Mass.cg_m
  Constant1 : Constant  Value=Aircraft.Geom.cp_m
  Mux : Mux  Inputs=2
  Terminator : Terminator
  Fxyz Mxyz : Outport
  wires:
  Mux/1 -> Fxyz Mxyz/1
  Constant1/1 -> "Aerodynamic Forces and Moments "/4
  Coef/1 -> "Aerodynamic Forces and Moments "/1
  Constant/1 -> "Aerodynamic Forces and Moments "/3
  "Aerodynamic Forces and Moments "/1 -> Mux/1
  "Aerodynamic Forces and Moments "/2 -> Mux/2
  Dynamic Pressure [Pa]/1 -> "Aerodynamic Forces and Moments "/2
  Body Velocity [m/s]/1 -> Terminator/1

== system trim_sim/Vehicle/Forces and Moments/Aerodynamic/Aerodynamic Forces and Moments Coef Axis Variant/Stability Axis Coef ==
  Coef : Inport
  Dynamic Pressure [Pa] : Inport  Port=2
  Body Velocity [m/s] : Inport  Port=3
  "Aerodynamic Forces and Moments " : aerolibadyn/Aerodynamic Forces and Moments   inputAxes=Stability  outputForceAxes=Body  outputMomentAxes=Body  S=Aircraft.Geom.s_m2  b=Aircraft.Geom.b_m  cbar=Aircraft.Geom.c_m
  Constant : Constant  Value=Aircraft.Mass.cg_m
  Constant1 : Constant  Value=Aircraft.Geom.cp_m
  Mux : Mux  Inputs=2
  Fxyz Mxyz : Outport
  wires:
  Dynamic Pressure [Pa]/1 -> "Aerodynamic Forces and Moments "/2
  "Aerodynamic Forces and Moments "/2 -> Mux/2
  "Aerodynamic Forces and Moments "/1 -> Mux/1
  Constant/1 -> "Aerodynamic Forces and Moments "/3
  Coef/1 -> "Aerodynamic Forces and Moments "/1
  Constant1/1 -> "Aerodynamic Forces and Moments "/4
  Mux/1 -> Fxyz Mxyz/1
  Body Velocity [m/s]/1 -> "Aerodynamic Forces and Moments "/5

== system trim_sim/Vehicle/Forces and Moments/Aerodynamic/Aerodynamic Forces and Moments Coef Axis Variant/Wind Axis Coef ==
  Coef : Inport
  Dynamic Pressure [Pa] : Inport  Port=2
  Body Velocity [m/s] : Inport  Port=3
  "Aerodynamic Forces and Moments " : aerolibadyn/Aerodynamic Forces and Moments   inputAxes=Wind  outputForceAxes=Body  outputMomentAxes=Body  S=Aircraft.Geom.s_m2  b=Aircraft.Geom.b_m  cbar=Aircraft.Geom.c_m
  Constant : Constant  Value=Aircraft.Mass.cg_m
  Constant1 : Constant  Value=Aircraft.Geom.cp_m
  Mux : Mux  Inputs=2
  Fxyz Mxyz : Outport
  wires:
  Dynamic Pressure [Pa]/1 -> "Aerodynamic Forces and Moments "/2
  Body Velocity [m/s]/1 -> "Aerodynamic Forces and Moments "/5
  "Aerodynamic Forces and Moments "/2 -> Mux/2
  "Aerodynamic Forces and Moments "/1 -> Mux/1
  Constant/1 -> "Aerodynamic Forces and Moments "/3
  Coef/1 -> "Aerodynamic Forces and Moments "/1
  Constant1/1 -> "Aerodynamic Forces and Moments "/4
  Mux/1 -> Fxyz Mxyz/1

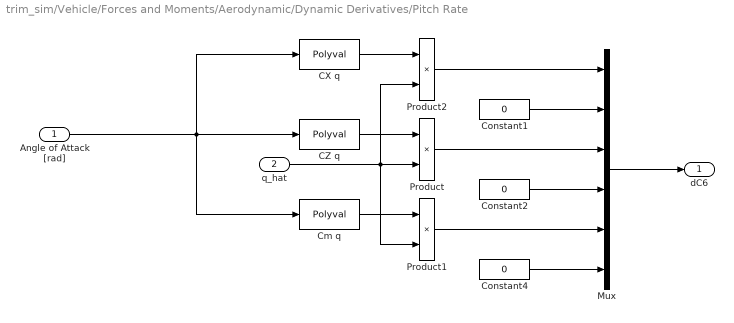
== system trim_sim/Vehicle/Forces and Moments/Aerodynamic/Dynamic Derivatives/Pitch Rate ==
  Angle of Attack [rad] : Inport
  q_hat : Inport  Port=2
  CX q : Polyval  Coefs=Aircraft.Aero.CX.q
  CZ q : Polyval  Coefs=Aircraft.Aero.CZ.q
  Cm q : Polyval  Coefs=Aircraft.Aero.Cm.q
  Constant1 : Constant  Value=0
  Constant2 : Constant  Value=0
  Constant4 : Constant  Value=0
  Mux : Mux  Inputs=6
  Product : Product
  Product1 : Product
  Product2 : Product
  dC6 : Outport
  wires:
  Mux/1 -> dC6/1
  Constant1/1 -> Mux/2
  Product2/1 -> Mux/1
  Constant4/1 -> Mux/6
  Constant2/1 -> Mux/4
  Product/1 -> Mux/3
  Product1/1 -> Mux/5
  q_hat/1 -> Product2/2, Product1/2, Product/2
  CZ q/1 -> Product/1
  CX q/1 -> Product2/1
  Cm q/1 -> Product1/1
  Angle of Attack [rad]/1 -> CX q/1, Cm q/1, CZ q/1

== system trim_sim/Vehicle/Forces and Moments/Aerodynamic/Dynamic Derivatives/Roll Rate ==
  Angle of Attack [rad] : Inport
  p_hat : Inport  Port=2
  CY p : Polyval  Coefs=Aircraft.Aero.CY.p
  Cl p : Polyval  Coefs=Aircraft.Aero.Cl.p
  Cn p : Polyval  Coefs=Aircraft.Aero.Cn.p
  Constant : Constant  Value=0
  Constant2 : Constant  Value=0
  Constant4 : Constant  Value=0
  Mux : Mux  Inputs=6
  Product : Product
  Product1 : Product
  Product2 : Product
  dC6 : Outport
  wires:
  Product1/1 -> Mux/4
  Product2/1 -> Mux/6
  Constant/1 -> Mux/1
  Mux/1 -> dC6/1
  Product/1 -> Mux/2
  CY p/1 -> Product/1
  Cl p/1 -> Product1/1
  Constant2/1 -> Mux/3
  Constant4/1 -> Mux/5
  p_hat/1 -> Product2/2, Product1/2, Product/2
  Cn p/1 -> Product2/1
  Angle of Attack [rad]/1 -> Cn p/1, CY p/1, Cl p/1

== system trim_sim/Vehicle/Forces and Moments/Aerodynamic/Dynamic Derivatives/Yaw Rate ==
  Angle of Attack [rad] : Inport
  r_hat : Inport  Port=2
  CY r : Polyval  Coefs=Aircraft.Aero.CY.r
  Cl r : Polyval  Coefs=Aircraft.Aero.Cl.r
  Cn r : Polyval  Coefs=Aircraft.Aero.Cn.r
  Constant : Constant  Value=0
  Constant2 : Constant  Value=0
  Constant4 : Constant  Value=0
  Mux : Mux  Inputs=6
  Product : Product
  Product1 : Product
  Product2 : Product
  dC6 : Outport
  wires:
  r_hat/1 -> Product2/2, Product1/2, Product/2
  Mux/1 -> dC6/1
  CY r/1 -> Product/1
  Constant/1 -> Mux/1
  Product2/1 -> Mux/6
  Product/1 -> Mux/2
  Cl r/1 -> Product1/1
  Constant2/1 -> Mux/3
  Product1/1 -> Mux/4
  Constant4/1 -> Mux/5
  Cn r/1 -> Product2/1
  Angle of Attack [rad]/1 -> Cn r/1, CY r/1, Cl r/1

== matlab function trim_sim/Vehicle/Vehicle Model/MATLAB Function ==
  data: ang input; ret output
function ret  = constrain360(ang)
%Constrain360 Converts a +/-180 value to a 0 - 360 value
ret = fmod(ang, 360);
if ret < 0
    ret = ret + 360;
end

end
